simulink model "example_trasmission"  (Simulink 9.0)
settings: Solver=ode45  StartTime=0.0  StopTime=2e-2  RelTol=1e-3
settings Model: Creator=CQC  LastModifiedBy=CQC
settings DataIOCC: SaveFormat=Dataset
settings OptimizationCC: LifeSpan=auto
settings DebuggingCC: UnderspecifiedInitializationDetection=Simplified  MergeDetectMultiDrivingBlocksExec=error  SFUnexpectedBacktrackingDiag=error  SFNoUnconditionalDefaultTransitionDiag=error  SFExecutionAtInitializationDiag=warning
settings HardwareCC: ProdBitPerPointer=64  ProdBitPerSizeT=64  ProdBitPerPtrDiffT=64  ProdLargestAtomicFloat=Float  ProdIntDivRoundTo=Zero  ProdEndianess=LittleEndian  ProdWordSize=64  ProdHWDeviceType=Intel->x86-64 (Windows64)
settings ModelReferenceCC: PropagateSignalLabelsOutOfModel=on
settings CodeAppCC: StateflowObjectComments=off
settings GRTTargetCC: TargetLangStandard=C99 (ISO)
settings ConfigComp: CovMetricSettings=dwe  CovHtmlReporting=off  CovSaveCumulativeToWorkspaceVar=off  CovSaveSingleToWorkspaceVar=off  CovExternalEMLEnable=on

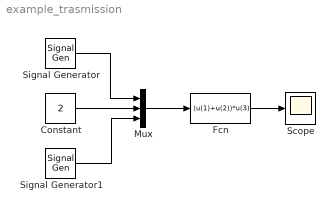
== system example_trasmission ==
  Constant : Constant  Value=2
  Fcn : Fcn  Expr=(u(1)+u(2))*u(3)
  Mux : Mux  Inputs=3
  Scope : Scope
  Signal Generator : SignalGenerator  Amplitude=2  Frequency=1000  Units=rad/sec
  Signal Generator1 : SignalGenerator  Amplitude=5  Frequency=1e4  Units=rad/sec
  wires:
  Signal Generator/1 -> Mux/1
  Constant/1 -> Mux/2
  Signal Generator1/1 -> Mux/3
  Mux/1 -> Fcn/1
  Fcn/1 -> Scope/1
